simulink library "Simple_lib"  (R2018b)
settings: Solver=ode45  StartTime=0.0  StopTime=10.0  RelTol=1e-3  EnableMultiTasking=on
undefined symbols (not defined in the file or in its folder): Acceptance, beta, C, C_J, C_P, c_wall, dGain, DiscIntNeverNeededParam, Duplex, Electrical_lib, grab, h_fe, i, i3, K_T, Kman, KmanCE, mu_s, n_rev, R_arm, Simplex, systemTs, tau_0, TinIC, Ts, w_0, wallMass, Watch_lib
libraries: $bdroot x407, PlantUtilityBlockset_lib x30, peGeneralControl x22, simulink x11
(part 8 of 14)

== system Simple_lib/Electronics/LR ==
  In1 : Inport
  In2 : Inport  Port=2
  1/R5 : Gain  Gain=-1
  Bus Creator : BusCreator  Inputs=3
  Bus Creator1 : BusCreator  Inputs=3
  Constant : Constant  Value=Phi_0
  Constant1 : Constant  Value=L
  Constant2 : Constant  Value=1/R
  Constant3 : Constant  Value=R
  Ground : Ground
  Ground1 : Ground
  Integrator (Discrete or Continuous) : peGeneralControl/Integrator (Discrete or Continuous)  LabelModeActiveChoice=Discrete  ExternalReset=level  LimitType=Anti-windup  B=inf  A=-inf  Ts=systemTs
  Max : MinMax  Function=max  Inputs=2
  Multiply : Product  Inputs=/*
  Resistance_in : Gain  Gain=R/2
  Resistance_out : Gain  Gain=R/2
  Sum : Sum  Inputs=-|+
  Sum2 : Sum  Inputs=|+-
  Sum3 : Sum  Inputs=|+-
  Weighted Sample Time2 : SampleTimeMath  TsampMathOp=*  weightValue=1
  _in : $bdroot/Electronics/_in  Level=V  Flow=I
      mask init:
      | initInput
      mask Display:
      | % This is a new mask on top of the base mask.
      | % Use "View base mask" link below to see the base mask.
      | %% Icon for flow in
      | % Signally design
      | %plot([0 2 2 3], [1 1 0 0])
      | %plot([1 3 2 1 0 2], [0.6 0.6 0.4 0.6 0.4 0.4])
      | %patch([1 3 2],[0.6 0.6 0.4])
      | %plot([0 1 1], [1 1 0.6])
      | %plot([1 1 0], [0.4 -1 -1])
      | 
      | %color('white')
      | %plot([0 3], [2 2])
      | %plot([0 3], [-2 -2])
      | 
      | %% Bolder design
      | %patch( [0 1 -1], [0 1 1])
      | patch( [-0.1 -0.1 -1], [0.95 0 0.95])
      | patch( [0.1 0.1 1], [1 0 1])
      | plot( [0.1 1 -1 -0.1], [0 -2 -2 0]*0.5)
      | %patch( [-0.1 0.1 0.1 -0.1], [0 0 1 1], [1 1 1])
      | %patch( [-1 0.1 0.1 -1], [1 1 0.95 0.95], [1 1 1])
      | 
      | %% Size the box
      | color('white')
      | plot( [-1 1], [2 2])
      | plot( [-1 1], -[2 2])
  _out : $bdroot/Electronics/_in  Level=V  Flow=I
      mask init:
      | initInput
      mask Display:
      | % This is a new mask on top of the base mask.
      | % Use "View base mask" link below to see the base mask.
      | %% Icon for flow in
      | % Signally design
      | %plot([0 2 2 3], [1 1 0 0])
      | %plot([1 3 2 1 0 2], [0.6 0.6 0.4 0.6 0.4 0.4])
      | %patch([1 3 2],[0.6 0.6 0.4])
      | %plot([0 1 1], [1 1 0.6])
      | %plot([1 1 0], [0.4 -1 -1])
      | 
      | %color('white')
      | %plot([0 3], [2 2])
      | %plot([0 3], [-2 -2])
      | 
      | %% Bolder design
      | %patch( [0 1 -1], [0 1 1])
      | patch( [-0.1 -0.1 -1], [0.95 0 0.95])
      | patch( [0.1 0.1 1], [1 0 1])
      | plot( [0.1 1 -1 -0.1], [0 -2 -2 0]*0.5)
      | %patch( [-0.1 0.1 0.1 -0.1], [0 0 1 1], [1 1 1])
      | %patch( [-1 0.1 0.1 -1], [1 1 0.95 0.95], [1 1 1])
      | 
      | %% Size the box
      | color('white')
      | plot( [-1 1], [2 2])
      | plot( [-1 1], -[2 2])
  wires:
  Weighted Sample Time2/1 -> Max/2  "L_min"
  Constant3/1 -> Weighted Sample Time2/1
  Constant1/1 -> Max/1
  Sum/1 -> Integrator (Discrete or Continuous)/1  "DV"
  Max/1 -> Multiply/1  "L"
  Multiply/1 -> Bus Creator/1, Resistance_out/1, 1/R5/1  "I"
  Bus Creator1/1 -> _in/2
  Bus Creator/1 -> _out/2
  Resistance_out/1 -> Sum3/2
  _out/1 -> Sum3/1
  In2/1 -> _out/1
  Integrator (Discrete or Continuous)/1 -> Multiply/2  "Phi"
  _in/1 -> Sum2/1
  Resistance_in/1 -> Sum2/2
  1/R5/1 -> Resistance_in/1, Bus Creator1/1  "I"
  In1/1 -> _in/1
  Sum2/1 -> Sum/1
  Sum3/1 -> Sum/2
  Constant2/1 -> Bus Creator1/3, Bus Creator/3  "G"
  Ground1/1 -> Bus Creator1/2, Bus Creator/2  "C"
  Constant/1 -> Integrator (Discrete or Continuous)/3
  Ground/1 -> Integrator (Discrete or Continuous)/2

== system Simple_lib/Electronics/M1 ==
  In1 : Inport
  _at : $bdroot/Electronics/_out  Tag=Electrical  Level=V  Flow=I
  _thru : $bdroot/Electronics/_in  Level=V  Flow=I
  Out1 : Outport
  wires:
  _at/1 -> Out1/1
  In1/1 -> _thru/1
  _thru/1 -> _at/1
  _at/2 -> _thru/2

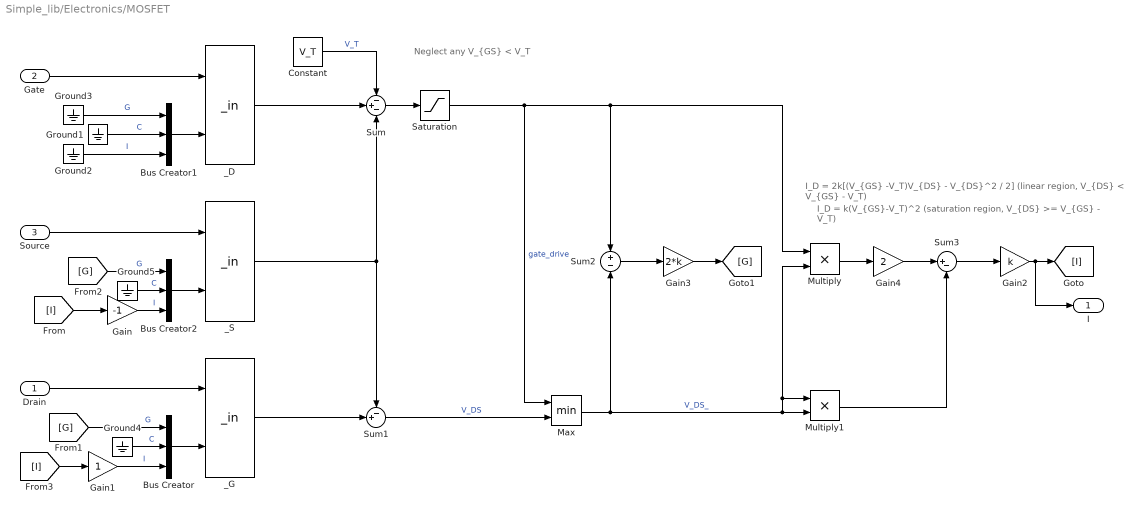
== system Simple_lib/Electronics/MOSFET ==
  note: Neglect any V_{GS} < V_T
  note: I_D = k(V_{GS}-V_T)^2 (saturation region, V_{DS} >= V_{GS} - V_T)
  note: I_D = 2k[(V_{GS} -V_T)V_{DS} - V_{DS}^2 / 2] (linear region, V_{DS} < V_{GS} - V_T)
  Drain : Inport
  Gate : Inport  Port=2
  Source : Inport  Port=3
  Bus Creator : BusCreator  Inputs=3
  Bus Creator1 : BusCreator  Inputs=3
  Bus Creator2 : BusCreator  Inputs=3
  Constant : Constant  Value=V_T
  Gain : Gain  Gain=-1
  Gain1 : Gain
  Gain2 : Gain  Gain=k
  Gain3 : Gain  Gain=2*k
  Gain4 : Gain  Gain=2
  Ground{1..5} (5 alike) : Ground
  Max : MinMax  Inputs=2
  Multiply : Product
  Multiply1 : Product
  Saturation : Saturate  UpperLimit=inf  LowerLimit=0
      settings: AttributesFormatString=|
      | %<UpperLimit>
      | %<LowerLimit>
  Sum : Sum  Inputs=-+-
  Sum1 : Sum  Inputs=-+|
  Sum2 : Sum  Inputs=+|-
  Sum3 : Sum  Inputs=|+-
  _D : $bdroot/Electronics/_in  Level=V  Flow=I
  _G : $bdroot/Electronics/_in  Level=V  Flow=I
  _S : $bdroot/Electronics/_in  Level=V  Flow=I
  I : Outport
  wires:
  Ground5/1 -> Bus Creator2/2  "C"
  Ground4/1 -> Bus Creator/2  "C"
  Gain2/1 -> I/1, [I]
  [I] -> Gain1/1
  [I] -> Gain/1
  [G] -> Bus Creator2/1  "G"
  [G] -> Bus Creator/1  "G"
  Sum3/1 -> Gain2/1
  Gain4/1 -> Sum3/1
  Multiply/1 -> Gain4/1
  Multiply1/1 -> Sum3/2
  Gain3/1 -> [G]
  Sum2/1 -> Gain3/1
  Max/1 -> Multiply/2, Multiply1/1, Multiply1/2, Sum2/2  "V_DS_"
  Sum1/1 -> Max/2  "V_DS"
  Saturation/1 -> Multiply/1, Sum2/1, Max/1  "gate_drive"
  Sum/1 -> Saturation/1
  Constant/1 -> Sum/1  "V_T"
  Ground2/1 -> Bus Creator1/3  "I"
  Gain/1 -> Bus Creator2/3  "I"
  Gain1/1 -> Bus Creator/3  "I"
  Ground3/1 -> Bus Creator1/1  "G"
  Bus Creator2/1 -> _S/2
  Bus Creator1/1 -> _D/2
  Ground1/1 -> Bus Creator1/2  "C"
  Bus Creator/1 -> _G/2
  Source/1 -> _S/1
  _G/1 -> Sum1/2
  _D/1 -> Sum/2
  Drain/1 -> _G/1
  _S/1 -> Sum1/1, Sum/3
  Gate/1 -> _D/1

== system Simple_lib/Electronics/MultiSource ==
  note: The Lump, from which the modelling technique got its name!
      | Lump together all the (grounded) capacitance and use this as inertia term in integrating I to get V.  Q = CV.
      | If there *isn't* much lumpable capacitance attached to this lump then estimate C, knowing R and Ts, by RC = Ts.
      | Integrate the sum of the currents divided by the sum of the grounded capacitances (lumped capacitance) to get the voltage.
      | If there is no capacitance, use Ts * lumped conductance.
  V_in : Inport
  V_in1 : Inport  Port=2
  Abs : Abs
  Abs1 : Abs
  Bus Selector : BusSelector  OutputSignals=I,G,C
  Constant1 : Constant  Value=1/2
  Detect Change : simulink/Logic and Bit Operations/Detect Change  vinit=0  OutDataTypeStr=boolean
  Divide1 : Product  Inputs=*/
  Ground : Ground
  Groundedness (Capacitance to ground) : Constant  Value=V_0
  Integrator (Discrete or Continuous) : peGeneralControl/Integrator (Discrete or Continuous)  LabelModeActiveChoice=Discrete  ExternalReset=level  LimitType=Anti-windup  B=inf  A=-inf  Ts=-1
  Max : MinMax  Function=max  Inputs=3
  Multiply1 : Product  Inputs=3
  Multiply2 : Product
  Saturation : Saturate  UpperLimit=slew_rate  LowerLimit=-slew_rate
      settings: AttributesFormatString=|
      | %<UpperLimit>
      | %<LowerLimit>
  Saturation1 : Saturate  UpperLimit=inf  LowerLimit=1e-12
  Sign convention : Gain  Gain=-1
  Sum : Sum  Inputs=++|
  Terminator1 : Terminator
  Terminator2 : Terminator
  Weighted Sample Time2 : SampleTimeMath  TsampMathOp=*  weightValue=1
  _out : $bdroot/Electronics/_out  Tag=Electrical  Level=V  Flow=I
  out : Outport
  wires:
  Sign convention/1 -> Sum/2  "Current fllow in"
  Saturation1/1 -> Divide1/2, Multiply2/2  "Ceff_sat"
  Integrator (Discrete or Continuous)/1 -> _out/1, Multiply1/1, Multiply2/1  "w"
  Multiply2/1 -> Multiply1/3, Terminator2/1  "conserved_quantity"
  Multiply1/1 -> Terminator1/1  "energy"
  Constant1/1 -> Multiply1/2
  Abs1/1 -> Max/1  "CestPos"
  Abs/1 -> Max/2  "Cpos"
  Sum/1 -> Divide1/1  "Current fllow in"
  Max/1 -> Saturation1/1  "Ceff"
  Weighted Sample Time2/1 -> Abs1/1  "Cest"
  Bus Selector/2 -> Weighted Sample Time2/1  "<G>"
  V_in/1 -> Detect Change/1, Integrator (Discrete or Continuous)/3
  Detect Change/1 -> Integrator (Discrete or Continuous)/2
  Bus Selector/3 -> Abs/1  "<C>"
  Bus Selector/1 -> Sign convention/1  "<I>"
  _out/2 -> Bus Selector/1
  _out/1 -> out/1
  Saturation/1 -> Integrator (Discrete or Continuous)/1  "dV"
  Divide1/1 -> Saturation/1
  Groundedness (Capacitance to ground)/1 -> Max/3
  V_in1/1 -> Sum/1

== system Simple_lib/Electronics/NPN ==
  note: D
  Collector : Inport
  Base : Inport  Port=2
  Emitter : Inport  Port=3
  Dbc : $bdroot/Electronics/D  I_S=1e-12  n=n  T_def=T_def
  Dbe : $bdroot/Electronics/D  I_S=I_S  n=n  T_def=T_def
  Isrc : $bdroot/Electronics/Isrc  SystemSampleTime=-1
  Isrc1 : $bdroot/Electronics/Isrc  SystemSampleTime=-1
  Sum : Sum  Inputs=++|
  Terminator : Terminator
  Terminator1 : Terminator
  alpha_F : Gain  Gain=alpha_F
  alpha_R : Gain  Gain=alpha_R
  I : Outport
  wires:
  Isrc/1 -> Terminator1/1
  Isrc1/1 -> Terminator/1
  Emitter/1 -> Isrc1/1, Dbe/3
  Collector/1 -> Dbc/3, Isrc/1
  Dbc/1 -> Sum/2, [I_BC]  "Icd"
  [I_BE] -> alpha_F/1
  alpha_F/1 -> Sum/1, Isrc/2
  [I_BC] -> alpha_R/1
  alpha_R/1 -> Isrc1/2
  Dbe/1 -> [I_BE]  "Ied"
  Base/1 -> Dbc/1, Isrc/3, Isrc1/3, Dbe/1
  Sum/1 -> I/1

== system Simple_lib/Electronics/NPN_RR ==
  note: D
  Collector : Inport
  Base : Inport  Port=2
  Emitter : Inport  Port=3
  D_Col : $bdroot/Electronics/D_RR  g=1e-3  V_drop=0.6
  D_Emt : $bdroot/Electronics/D_RR  g=1e-3  V_drop=0.6
  Src_Col : $bdroot/Electronics/Isrc  SystemSampleTime=-1
  Src_Emt : $bdroot/Electronics/Isrc  SystemSampleTime=-1
  Terminator : Terminator
  Terminator1 : Terminator
  alpha_F : Gain  Gain=alpha_F
  alpha_R : Gain  Gain=alpha_R
  wires:
  Src_Col/1 -> Terminator1/1
  Src_Emt/1 -> Terminator/1
  Emitter/1 -> D_Emt/2, Src_Emt/1
  Collector/1 -> D_Col/2, Src_Col/1
  D_Col/1 -> [I_CD]  "Icd"
  [I_ED] -> alpha_F/1
  alpha_F/1 -> Src_Col/2
  [I_CD] -> alpha_R/1
  alpha_R/1 -> Src_Emt/2
  D_Emt/1 -> [I_ED]  "Ied"
  Base/1 -> D_Emt/1, D_Col/1, Src_Col/3, Src_Emt/3

== system Simple_lib/Electronics/NPN_SimpleRR ==
  Collector : Inport
  Base : Inport  Port=2
  Emitter : Inport  Port=3
  D_be : $bdroot/Electronics/D_  g_on=0.001  g_off=1e-5  V_drop=1.4
  TransistorMan : Subsystem  mask{V_drop=.6}
      mask prompts: V_drop "Potential Drop (V)"
      mask Display:
      | %patch( [0 -0.05 -0.05 0],[-1 -1 1 1])
      | %patch( [0 1 1],[0 1 -1])
  wires:
  D_be/1 -> TransistorMan/2(I)
  Base/1 -> D_be/1
  Emitter/1 -> TransistorMan/3(Emitter), D_be/2
  Collector/1 -> TransistorMan/1(Collector)

== system Simple_lib/Electronics/OpAmp ==
  note: Just want 1/Ts as the gain, irrespective of the current stuff. I think.
  + : Inport
  - : Inport  Port=2
  Bus Creator1 : BusCreator  Inputs=3
  Ground{,1..4} (5 alike) : Ground
  Integrator (Discrete or Continuous) : peGeneralControl/Integrator (Discrete or Continuous)  LabelModeActiveChoice=Discrete  ExternalReset=level  LimitType=Anti-windup  B=inf  A=-inf  Ts=-1
  Sum : Sum  Inputs=+|-
  Terminator : Terminator
  Weighted Sample Time2 : SampleTimeMath  TsampMathOp=/  weightValue=1
  _out : $bdroot/Electronics/_out  Tag=Electrical  Level=V  Flow=I
  neg : $bdroot/Electronics/OpAmp/pos
      mask init:
      | initInput
      mask Display:
      | % This is a new mask on top of the base mask.
      | % Use "View base mask" link below to see the base mask.
      | %% Icon for flow in
      | % Signally design
      | %plot([0 2 2 3], [1 1 0 0])
      | %plot([1 3 2 1 0 2], [0.6 0.6 0.4 0.6 0.4 0.4])
      | %patch([1 3 2],[0.6 0.6 0.4])
      | %plot([0 1 1], [1 1 0.6])
      | %plot([1 1 0], [0.4 -1 -1])
      | 
      | %color('white')
      | %plot([0 3], [2 2])
      | %plot([0 3], [-2 -2])
      | 
      | %% Bolder design
      | %patch( [0 1 -1], [0 1 1])
      | patch( [-0.1 -0.1 -1], [0.95 0 0.95])
      | patch( [0.1 0.1 1], [1 0 1])
      | plot( [0.1 1 -1 -0.1], [0 -2 -2 0]*0.5)
      | %patch( [-0.1 0.1 0.1 -0.1], [0 0 1 1], [1 1 1])
      | %patch( [-1 0.1 0.1 -1], [1 1 0.95 0.95], [1 1 1])
      | 
      | %% Size the box
      | color('white')
      | plot( [-1 1], [2 2])
      | plot( [-1 1], -[2 2])
  pos : $bdroot/Electronics/_in  Level=V  Flow=I
      mask init:
      | initInput
      mask Display:
      | % This is a new mask on top of the base mask.
      | % Use "View base mask" link below to see the base mask.
      | %% Icon for flow in
      | % Signally design
      | %plot([0 2 2 3], [1 1 0 0])
      | %plot([1 3 2 1 0 2], [0.6 0.6 0.4 0.6 0.4 0.4])
      | %patch([1 3 2],[0.6 0.6 0.4])
      | %plot([0 1 1], [1 1 0.6])
      | %plot([1 1 0], [0.4 -1 -1])
      | 
      | %color('white')
      | %plot([0 3], [2 2])
      | %plot([0 3], [-2 -2])
      | 
      | %% Bolder design
      | %patch( [0 1 -1], [0 1 1])
      | patch( [-0.1 -0.1 -1], [0.95 0 0.95])
      | patch( [0.1 0.1 1], [1 0 1])
      | plot( [0.1 1 -1 -0.1], [0 -2 -2 0]*0.5)
      | %patch( [-0.1 0.1 0.1 -0.1], [0 0 1 1], [1 1 1])
      | %patch( [-1 0.1 0.1 -1], [1 1 0.95 0.95], [1 1 1])
      | 
      | %% Size the box
      | color('white')
      | plot( [-1 1], [2 2])
      | plot( [-1 1], -[2 2])
  Out1 : Outport
  wires:
  _out/2 -> Terminator/1
  Ground2/1 -> Integrator (Discrete or Continuous)/3
  Ground/1 -> Integrator (Discrete or Continuous)/2
  pos/1 -> Sum/1
  neg/1 -> Sum/2
  +/1 -> pos/1
  -/1 -> neg/1
  _out/1 -> Out1/1
  Sum/1 -> Weighted Sample Time2/1
  Integrator (Discrete or Continuous)/1 -> _out/1
  Weighted Sample Time2/1 -> Integrator (Discrete or Continuous)/1
  Bus Creator1/1 -> neg/2, pos/2
  Ground4/1 -> Bus Creator1/2  "C"
  Ground3/1 -> Bus Creator1/1  "I"
  Ground1/1 -> Bus Creator1/3  "G"

== system Simple_lib/Electronics/PNP ==
  note: D
  Collector : Inport
  Base : Inport  Port=2
  Emitter : Inport  Port=3
  Dbc : $bdroot/Electronics/D  I_S=1e-12  n=1  T_def=300
  Dbe : $bdroot/Electronics/D  I_S=1e-12  n=1  T_def=300
  Isrc : $bdroot/Electronics/Isrc  SystemSampleTime=-1
  Isrc1 : $bdroot/Electronics/Isrc  SystemSampleTime=-1
  Sum : Sum  Inputs=++|
  Terminator : Terminator
  Terminator1 : Terminator
  alpha_F : Gain  Gain=alpha_F
  alpha_R : Gain  Gain=alpha_R
  I : Outport
  wires:
  Isrc1/1 -> Terminator1/1
  Isrc/1 -> Terminator/1
  Emitter/1 -> Dbe/1, Isrc/3
  Collector/1 -> Isrc1/3, Dbc/1
  [I_EB] -> alpha_F/1
  [I_CB] -> alpha_R/1
  alpha_R/1 -> Isrc/2
  Dbe/1 -> [I_EB]  "Ied"
  Base/1 -> Dbc/3, Dbe/3, Isrc1/1, Isrc/1
  Dbc/1 -> Sum/2, [I_CB]  "Icd"
  alpha_F/1 -> Isrc1/2, Sum/1
  Sum/1 -> I/1

== system Simple_lib/Electronics/PNP_RR ==
  note: D
  Collector : Inport
  Base : Inport  Port=2
  Emitter : Inport  Port=3
  D_bc : $bdroot/Electronics/D_RR  g=1e-3  V_drop=0.6
  D_be : $bdroot/Electronics/D_RR  g=1e-3  V_drop=0.6
  Isrc : $bdroot/Electronics/Isrc  SystemSampleTime=-1
  Isrc1 : $bdroot/Electronics/Isrc  SystemSampleTime=-1
  Terminator : Terminator
  Terminator1 : Terminator
  alpha_F : Gain  Gain=alpha_F
  alpha_R : Gain  Gain=alpha_R
  wires:
  Isrc1/1 -> Terminator1/1
  Isrc/1 -> Terminator/1
  Emitter/1 -> D_be/1, Isrc/3
  Collector/1 -> D_bc/1, Isrc1/3
  D_bc/1 -> [I_CD]  "Icd"
  [I_ED] -> alpha_F/1
  alpha_F/1 -> Isrc1/2
  [I_CD] -> alpha_R/1
  alpha_R/1 -> Isrc/2
  D_be/1 -> [I_ED]  "Ied"
  Base/1 -> D_bc/2, D_be/2, Isrc1/1, Isrc/1

== system Simple_lib/Electronics/Q ==
  Collector : Inport
  Emitter : Inport  Port=2
  Diode : $bdroot/Electronics/Reverse  V_drop=0
  Sum : Sum  Inputs=+|+
  TransAction : $bdroot/Electronics/TransAction  V_drop=.6
  Base : Outport
  wires:
  TransAction/1 -> Sum/1
  Sum/1 -> Base/1
  Collector/1 -> TransAction/1
  Emitter/1 -> Diode/1
  Diode/1 -> TransAction/2, Sum/2

== system Simple_lib/Electronics/Q1 ==
  note: D
  Collector : Inport
  Base : Inport  Port=2
  Emitter : Inport  Port=3
  Dc : $bdroot/Electronics/D_  g_on=g_on  g_off=g_off  V_drop=V_drop
  De : $bdroot/Electronics/D_  g_on=1e-1  g_off=0  V_drop=0.6
  Ic : $bdroot/Electronics/Isrc  SystemSampleTime=-1
  Ie : $bdroot/Electronics/Isrc  SystemSampleTime=-1
  Terminator : Terminator
  Terminator1 : Terminator
  alpha_F : Gain  Gain=alpha_F
  alpha_R : Gain  Gain=alpha_R
  wires:
  Base/1 -> De/1, Dc/1, Ie/3, Ic/3
  De/1 -> alpha_F/1  "Ied"
  alpha_R/1 -> Ie/2
  alpha_F/1 -> Ic/2
  Dc/1 -> alpha_R/1  "Icd"
  Collector/1 -> Dc/2, Ic/1
  Emitter/1 -> De/2, Ie/1
  Ie/1 -> Terminator/1
  Ic/1 -> Terminator1/1

== system Simple_lib/Electronics/Q2 ==
  note: D
  Collector : Inport
  Base : Inport  Port=2
  Emitter : Inport  Port=3
  Dc : $bdroot/Electronics/D_  g_on=0.001  g_off=1e-5  V_drop=V_drop
  De : $bdroot/Electronics/D_  g_on=0.001  g_off=1e-5  V_drop=V_drop
  Isrc : $bdroot/Electronics/Isrc  SystemSampleTime=-1
  Isrc1 : $bdroot/Electronics/Isrc  SystemSampleTime=-1
  Terminator : Terminator
  Terminator1 : Terminator
  alpha_F : Gain  Gain=alpha_F
  alpha_R : Gain  Gain=alpha_R
  wires:
  Isrc1/1 -> Terminator1/1
  Isrc/1 -> Terminator/1
  Emitter/1 -> De/1, Isrc/3
  Collector/1 -> Dc/1, Isrc1/3
  Dc/1 -> alpha_R/1  "Icd"
  alpha_F/1 -> Isrc1/2
  alpha_R/1 -> Isrc/2
  De/1 -> alpha_F/1  "Ied"
  Base/1 -> De/2, Dc/2, Isrc1/1, Isrc/1

== system Simple_lib/Electronics/Q_NPN ==
  note: D
  Base : Inport
  Ammeter : $bdroot/Electronics/Ammeter  SystemSampleTime=-1
  Ammeter1 : $bdroot/Electronics/Ammeter  SystemSampleTime=-1
  Dbc : $bdroot/Electronics/Forward  V_drop=0.6
  Dbe : $bdroot/Electronics/Forward  V_drop=0.6
  SrcCb : $bdroot/Electronics/Isrc  SystemSampleTime=-1
  SrcEb : $bdroot/Electronics/Isrc  SystemSampleTime=-1
  Sum : Sum  Inputs=++|
  Sum1 : Sum  Inputs=++|
  Terminator : Terminator
  Terminator1 : Terminator
  Unit Delay1 : UnitDelay  SampleTime=-1
  Unit Delay2 : UnitDelay  Commented=through  SampleTime=-1
  alpha_F : Gain  Gain=alpha_F
  alpha_R : Gain  Gain=alpha_R
  C : Outport
  E : Outport  Port=2
  wires:
  Unit Delay2/1 -> SrcEb/2
  Unit Delay1/1 -> SrcCb/2
  alpha_R/1 -> Unit Delay2/1
  Ammeter1/1 -> Sum/1
  Ammeter/1 -> Sum1/1
  Dbe/1 -> Sum/2
  Dbc/1 -> Sum1/2
  Base/1 -> Dbc/1, Dbe/1, SrcCb/3, SrcEb/3
  SrcCb/1 -> Terminator1/1
  SrcEb/1 -> Terminator/1
  Sum/1 -> E/1, SrcEb/1
  Sum1/1 -> SrcCb/1, C/1
  Ammeter/2 -> alpha_R/1  "Ibc"
  alpha_F/1 -> Unit Delay1/1
  Ammeter1/2 -> alpha_F/1  "Ibe"

== system Simple_lib/Electronics/R ==
  pos : Inport
  neg : Inport  Port=2
  1/R1 : Gain  Gain=-1
  Bus Creator : BusCreator  Inputs=3
  Bus Creator1 : BusCreator  Inputs=3
  Constant1 : Constant  Value=1/R
  Ground : Ground
  Sum : Sum  Inputs=+|-
  _neg : $bdroot/Electronics/_in  Level=V  Flow=I
  _pos : $bdroot/Electronics/_in  Level=V  Flow=I
  conductance1 : Gain  Gain=1/R
  I : Outport
  wires:
  _neg/1 -> Sum/2
  1/R1/1 -> Bus Creator1/3  "I"
  conductance1/1 -> Bus Creator/1, I/1, 1/R1/1  "I"
  Bus Creator/1 -> _pos/2
  Sum/1 -> conductance1/1
  Bus Creator1/1 -> _neg/2
  _pos/1 -> Sum/1
  pos/1 -> _pos/1
  neg/1 -> _neg/1
  Constant1/1 -> Bus Creator/2, Bus Creator1/2  "G"
  Ground/1 -> Bus Creator1/1, Bus Creator/3  "C"

== system Simple_lib/Electronics/R1 ==
  pos : Inport
  neg : Inport  Port=2
  1/R1 : Gain  Gain=-1
  Bus Creator : BusCreator  Inputs=3
  Bus Creator1 : BusCreator  Inputs=3
  Constant1 : Constant  Value=1/R
  Ground : Ground
  Sum : Sum  Inputs=+|-
  _neg : $bdroot/Electronics/_in  Level=V  Flow=I
  _pos : $bdroot/Electronics/_in  Level=V  Flow=I
  conductance1 : Gain  Gain=1/R
  I : Outport
  wires:
  _neg/1 -> Sum/2
  1/R1/1 -> Bus Creator1/3  "I"
  conductance1/1 -> Bus Creator/1, I/1, 1/R1/1  "I"
  Bus Creator/1 -> _pos/2
  Sum/1 -> conductance1/1
  Bus Creator1/1 -> _neg/2
  _pos/1 -> Sum/1
  pos/1 -> _pos/1
  neg/1 -> _neg/1
  Constant1/1 -> Bus Creator/2, Bus Creator1/2  "G"
  Ground/1 -> Bus Creator1/1, Bus Creator/3  "C"

== system Simple_lib/Electronics/R_ ==
  In1 : Inport
  Ground1 : Ground
  at : $bdroot/Electronics/TP  V_0=0  slew_rate=1000  conserved_quantity_name=Q  energy_name=E
  thru : $bdroot/Electronics/R  R=R
      settings: AttributesFormatString=%<R> Ohms
  Out1 : Outport
  wires:
  In1/1 -> thru/1
  at/1 -> thru/2, Out1/1
  Ground1/1 -> at/1

== system Simple_lib/Electronics/R_1 ==
  In1 : Inport
  Bus Selector : BusSelector  OutputSignals=I
  In : $bdroot/Electronics/_in  Level=V  Flow=I
      mask init:
      | initInput
      mask Display:
      | % This is a new mask on top of the base mask.
      | % Use "View base mask" link below to see the base mask.
      | %% Icon for flow in
      | % Signally design
      | %plot([0 2 2 3], [1 1 0 0])
      | %plot([1 3 2 1 0 2], [0.6 0.6 0.4 0.6 0.4 0.4])
      | %patch([1 3 2],[0.6 0.6 0.4])
      | %plot([0 1 1], [1 1 0.6])
      | %plot([1 1 0], [0.4 -1 -1])
      | 
      | %color('white')
      | %plot([0 3], [2 2])
      | %plot([0 3], [-2 -2])
      | 
      | %% Bolder design
      | %patch( [0 1 -1], [0 1 1])
      | patch( [-0.1 -0.1 -1], [0.95 0 0.95])
      | patch( [0.1 0.1 1], [1 0 1])
      | plot( [0.1 1 -1 -0.1], [0 -2 -2 0]*0.5)
      | %patch( [-0.1 0.1 0.1 -0.1], [0 0 1 1], [1 1 1])
      | %patch( [-1 0.1 0.1 -1], [1 1 0.95 0.95], [1 1 1])
      | 
      | %% Size the box
      | color('white')
      | plot( [-1 1], [2 2])
      | plot( [-1 1], -[2 2])
  Sum : Sum  Inputs=|+-
  _out : $bdroot/Electronics/_out  Tag=Electrical  Level=V  Flow=I
  resistance : Gain  Gain=R
  Out1 : Outport
  wires:
  In/1 -> Sum/1
  _out/2 -> In/2, Bus Selector/1
  resistance/1 -> Sum/2
  Sum/1 -> _out/1
  _out/1 -> Out1/1
  In1/1 -> In/1
  Bus Selector/1 -> resistance/1  "<I>"

== system Simple_lib/Electronics/R_Gnd ==
  In1 : Inport
  Gnd : $bdroot/Electronics/Earth  SystemSampleTime=-1
  at : $bdroot/Electronics/R  R=R
      settings: AttributesFormatString=%<R> Ohms
  wires:
  In1/1 -> at/1
  Gnd/1 -> at/2

== system Simple_lib/Electronics/Rail ==
  V : Inport
  Bus Selector : BusSelector  OutputSignals=I
  Constant : Constant  Value=Vcc
  Sum : Sum  Inputs=|++
  _in : $bdroot/Electronics/_out  Tag=Electrical  Level=V  Flow=I
  I : Outport
  Vcc : Outport  Port=2
  wires:
  _in/1 -> Vcc/1
  Constant/1 -> Sum/2
  _in/2 -> Bus Selector/1
  Bus Selector/1 -> I/1  "<I>"
  Sum/1 -> _in/1
  V/1 -> Sum/1

== system Simple_lib/Electronics/ResistiveSwitch ==
  s : Inport
  In2 : Inport  Port=2
  Switch : $bdroot/Electronics/Switch  SystemSampleTime=-1
  from : $bdroot/Electronics/TP  V_0=0  slew_rate=100.0  conserved_quantity_name=Q  energy_name=E
  Out1 : Outport
  wires:
  In2/1 -> Switch/3
  from/1 -> Switch/1, Out1/1
  s/1 -> Switch/2

== system Simple_lib/Electronics/Reverse ==
  in : Inport
  Bus Creator2 : BusCreator  Inputs=3
  Bus Selector : BusSelector  OutputSignals=I,C,G
  Bus Selector1 : BusSelector  OutputSignals=I,C,G
  Constant : Constant  Value=-V_drop
  Divide1 : Product  Inputs=*/
  Gain : Gain
  Gain1 : Gain
  Ground : Ground
  Ground1 : Ground  Commented=on
  Integrator (Discrete or Continuous) : peGeneralControl/Integrator (Discrete or Continuous)  LabelModeActiveChoice=Discrete  ExternalReset=level  LimitType=Anti-windup  B=inf  A=-V_drop  Ts=systemTs
  Sum1 : Sum  Inputs=|+-
  Switch : Switch  Criteria=u2 ~= 0
  Weighted Sample Time : SampleTimeMath  TsampMathOp=*
  _in : $bdroot/Electronics/_in  Level=V  Flow=I
  _out : $bdroot/Electronics/_out  Tag=Electrical  Level=V  Flow=I
  out : Outport
  wires:
  Bus Creator2/1 -> _in/2
  Gain1/1 -> Bus Creator2/2  "C"
  Gain/1 -> Bus Creator2/3  "G"
  Bus Selector1/3 -> Gain/1  "<G>"
  Bus Selector1/2 -> Gain1/1  "<C>"
  Bus Selector1/1 -> Bus Creator2/1  "<I>"
  Ground1/1 -> ?  "I"
  _out/1 -> out/1
  Integrator (Discrete or Continuous)/1 -> Sum1/2
  _in/1 -> Sum1/1
  in/1 -> _in/1
  Sum1/1 -> _out/1
  Bus Selector/2 -> Switch/1, Switch/2  "<C>"
  Bus Selector/1 -> Divide1/1  "<I>"
  Divide1/1 -> Integrator (Discrete or Continuous)/1
  Constant/1 -> Integrator (Discrete or Continuous)/3
  Ground/1 -> Integrator (Discrete or Continuous)/2
  _out/2 -> Bus Selector/1, Bus Selector1/1
  Weighted Sample Time/1 -> Switch/3
  Bus Selector/3 -> Weighted Sample Time/1  "<G>"
  Switch/1 -> Divide1/2

== system Simple_lib/Electronics/Rnl1 ==
  note: Put the exponential terms from Ebers Moll in here - the Shockley model
  pos : Inport
  neg : Inport  Port=2
  1/R1 : Gain  Gain=-1
  Bus Creator : BusCreator  Inputs=3
  Bus Creator1 : BusCreator  Inputs=3
  Derivative : Subsystem
  Ground : Ground
  I/V curve : Lookup_n-D  Commented=on  NumberOfTableDimensions=1  BreakpointsForDimension1=[-5:5]  Table=tanh([-5:5])  InternalRulePriority=Speed  RndMeth=Simplest  InputSameDT=on
  I/V curve1 : Lookup_n-D  NumberOfTableDimensions=1  BreakpointsForDimension1=[-5:5]  Table=[0 0 0 0 0 0 0 1 10 100 1000]  InternalRulePriority=Speed  RndMeth=Simplest  InputSameDT=on
  Sum : Sum  Inputs=+|-
  _neg : $bdroot/Electronics/_in  Level=V  Flow=I
      mask init:
      | initInput
      mask Display:
      | % This is a new mask on top of the base mask.
      | % Use "View base mask" link below to see the base mask.
      | %% Icon for flow in
      | % Signally design
      | %plot([0 2 2 3], [1 1 0 0])
      | %plot([1 3 2 1 0 2], [0.6 0.6 0.4 0.6 0.4 0.4])
      | %patch([1 3 2],[0.6 0.6 0.4])
      | %plot([0 1 1], [1 1 0.6])
      | %plot([1 1 0], [0.4 -1 -1])
      | 
      | %color('white')
      | %plot([0 3], [2 2])
      | %plot([0 3], [-2 -2])
      | 
      | %% Bolder design
      | %patch( [0 1 -1], [0 1 1])
      | patch( [-0.1 -0.1 -1], [0.95 0 0.95])
      | patch( [0.1 0.1 1], [1 0 1])
      | plot( [0.1 1 -1 -0.1], [0 -2 -2 0]*0.5)
      | %patch( [-0.1 0.1 0.1 -0.1], [0 0 1 1], [1 1 1])
      | %patch( [-1 0.1 0.1 -1], [1 1 0.95 0.95], [1 1 1])
      | 
      | %% Size the box
      | color('white')
      | plot( [-1 1], [2 2])
      | plot( [-1 1], -[2 2])
  _pos : $bdroot/Electronics/_in  Level=V  Flow=I
      mask init:
      | initInput
      mask Display:
      | % This is a new mask on top of the base mask.
      | % Use "View base mask" link below to see the base mask.
      | %% Icon for flow in
      | % Signally design
      | %plot([0 2 2 3], [1 1 0 0])
      | %plot([1 3 2 1 0 2], [0.6 0.6 0.4 0.6 0.4 0.4])
      | %patch([1 3 2],[0.6 0.6 0.4])
      | %plot([0 1 1], [1 1 0.6])
      | %plot([1 1 0], [0.4 -1 -1])
      | 
      | %color('white')
      | %plot([0 3], [2 2])
      | %plot([0 3], [-2 -2])
      | 
      | %% Bolder design
      | %patch( [0 1 -1], [0 1 1])
      | patch( [-0.1 -0.1 -1], [0.95 0 0.95])
      | patch( [0.1 0.1 1], [1 0 1])
      | plot( [0.1 1 -1 -0.1], [0 -2 -2 0]*0.5)
      | %patch( [-0.1 0.1 0.1 -0.1], [0 0 1 1], [1 1 1])
      | %patch( [-1 0.1 0.1 -1], [1 1 0.95 0.95], [1 1 1])
      | 
      | %% Size the box
      | color('white')
      | plot( [-1 1], [2 2])
      | plot( [-1 1], -[2 2])
  I : Outport
  wires:
  1/R1/1 -> Bus Creator1/2  "I"
  Bus Creator/1 -> _pos/2
  Derivative/1(dy/dx) -> Bus Creator/1, Bus Creator1/3  "G"
  pos/1 -> _pos/1
  _pos/1 -> Sum/1
  Sum/1 -> I/V curve1/1, Derivative/2(x)  "D_V"
  neg/1 -> _neg/1
  _neg/1 -> Sum/2
  I/V curve1/1 -> I/1, 1/R1/1, Bus Creator/2, Derivative/1(y)  "I"
  Bus Creator1/1 -> _neg/2
  Ground/1 -> Bus Creator/3, Bus Creator1/1  "C"

== system Simple_lib/Electronics/Switch ==
  In1 : Inport
  In2 : Inport  Port=2
  In3 : Inport  Port=3
  Switch : Switch  Criteria=u2 ~= 0
  VR : $bdroot/Electronics/VR  SystemSampleTime=-1
  g_off : Constant  Value=10e-9
  g_on : Constant  Value=100
  wires:
  In2/1 -> Switch/2
  In3/1 -> VR/3
  In1/1 -> VR/1
  Switch/1 -> VR/2
  g_on/1 -> Switch/1
  g_off/1 -> Switch/3

== system Simple_lib/Electronics/Switch2 ==
  In1 : Inport
  In2 : Inport  Port=2
  In3 : Inport  Port=3
  Ground : Ground
  Ground1 : Ground
  Switch : Switch  Criteria=u2 ~= 0
  Switch1 : Switch  Criteria=u2 ~= 0
  Switch2 : Switch  Criteria=u2 ~= 0
  _in1 : $bdroot/Electronics/_in  Level=V  Flow=I
  _in2 : $bdroot/Electronics/_in  Level=V  Flow=I
  _out : $bdroot/Electronics/_out  Tag=Electrical  Level=V  Flow=I
  Output : Outport
  wires:
  In2/1 -> Switch1/2, Switch2/2, Switch/2
  In3/1 -> _in2/1
  In1/1 -> _in1/1
  Switch/1 -> _out/1
  _in1/1 -> Switch/1
  _in2/1 -> Switch/3
  _out/1 -> Output/1
  _out/2 -> [I]
  Switch2/1 -> _in2/2
  Switch1/1 -> _in1/2
  [I] -> Switch1/1
  [I] -> Switch2/3
  Ground1/1 -> Switch2/1
  Ground/1 -> Switch1/3

== system Simple_lib/Electronics/TP ==
  note: The Lump, from which the modelling technique got its name!
      | Lump together all the (grounded) capacitance and use this as inertia term in integrating I to get V.  Q = CV.
      | If there *isn't* much lumpable capacitance attached to this lump then estimate C, knowing R and Ts, by RC = Ts.
      | Integrate the sum of the currents divided by the sum of the grounded capacitances (lumped capacitance) to get the voltage.
      | If there is no capacitance, use Ts * lumped conductance.
  I : Inport
  Abs : Abs
  Abs1 : Abs
  Bus Selector : BusSelector  OutputSignals=I,G,C
  Constant : Constant  Value=V_0
  Constant1 : Constant  Value=1/2
  Divide1 : Product  Inputs=*/
  Ground : Ground
  Integrator (Discrete or Continuous) : peGeneralControl/Integrator (Discrete or Continuous)  LabelModeActiveChoice=Discrete  ExternalReset=level  LimitType=Anti-windup  B=inf  A=-inf  Ts=-1
  Max : MinMax  Function=max  Inputs=2
  Multiply1 : Product  Inputs=3
  Multiply2 : Product
  Saturation : Saturate  UpperLimit=slew_rate  LowerLimit=-slew_rate
      settings: AttributesFormatString=|
      | %<UpperLimit>
      | %<LowerLimit>
  Saturation1 : Saturate  UpperLimit=inf  LowerLimit=1e-12
  Sign convention : Gain  Gain=-1
  Sum : Sum  Inputs=++|
  Terminator1 : Terminator
  Terminator2 : Terminator
  Weighted Sample Time2 : SampleTimeMath  TsampMathOp=*  weightValue=1
  _out : $bdroot/Electronics/_out  Tag=Electrical  Level=V  Flow=I
  out : Outport
  wires:
  Divide1/1 -> Saturation/1
  Saturation/1 -> Integrator (Discrete or Continuous)/1  "dV"
  _out/1 -> out/1
  _out/2 -> Bus Selector/1
  Bus Selector/1 -> Sign convention/1  "<I>"
  Bus Selector/3 -> Abs/1  "C"
  Ground/1 -> Integrator (Discrete or Continuous)/2
  Constant/1 -> Integrator (Discrete or Continuous)/3
  Bus Selector/2 -> Weighted Sample Time2/1  "<G>"
  Weighted Sample Time2/1 -> Abs1/1  "Cest"
  Max/1 -> Saturation1/1  "Ceff"
  Sum/1 -> Divide1/1  "Current fllow in"
  Abs/1 -> Max/2  "Cpos"
  Abs1/1 -> Max/1  "CestPos"
  Constant1/1 -> Multiply1/2
  Multiply1/1 -> Terminator1/1  "energy"
  Multiply2/1 -> Terminator2/1, Multiply1/3  "conserved_quantity"
  Integrator (Discrete or Continuous)/1 -> Multiply2/1, Multiply1/1, _out/1  "w"
  Saturation1/1 -> Multiply2/2, Divide1/2  "Jeff_sat"
  I/1 -> Sum/1
  Sign convention/1 -> Sum/2  "Current fllow in"

== system Simple_lib/Electronics/TransAction ==
  Collector : Inport
  Emitter : Inport  Port=2
  Bus Creator : BusCreator  Inputs=3
  Bus Creator1 : BusCreator  Inputs=3
  Bus Selector : BusSelector  OutputSignals=I
  Constant : Constant  Value=99
  Constant1 : Constant  Value=99
  Cosh : Trigonometry  Operator=cosh
  Gain : Gain  Gain=-1
  Gain1 : Gain  Gain=-1
  Gain2 : Gain
  Gain3 : Gain
  Ground : Ground
  Ground1 : Ground
  Multiply : Product  Inputs=3
  Multiply1 : Product  Inputs=*//*
  Saturation : Saturate  UpperLimit=inf  LowerLimit=-inf
  Sum : Sum  Inputs=+|-
  Tanh : Trigonometry  Operator=tanh
  _Base : $bdroot/Electronics/_out  Tag=Electrical  Level=V  Flow=I
  _Col : $bdroot/Electronics/_in  Level=V  Flow=I
  _Em : $bdroot/Electronics/_in  Level=V  Flow=I
  Dummy : Outport
  wires:
  Gain3/1 -> Bus Creator/1  "I"
  Gain2/1 -> Bus Creator1/2  "G"
  Gain1/1 -> Saturation/1  "I"
  Saturation/1 -> Multiply/1, Multiply1/4
  Bus Selector/1 -> Gain1/1  "<I>"
  Constant1/1 -> Multiply1/1
  Multiply1/1 -> Bus Creator/2, Gain2/1  "G"
  Cosh/1 -> Multiply1/3, Multiply1/2
  Bus Creator/1 -> _Col/2
  Bus Creator1/1 -> _Em/2
  Ground1/1 -> Bus Creator/3, Bus Creator1/1  "C"
  Gain/1 -> Bus Creator1/3  "I"
  Multiply/1 -> Gain/1, Gain3/1  "I"
  Constant/1 -> Multiply/3
  _Base/2 -> Bus Selector/1
  Tanh/1 -> Multiply/2
  Sum/1 -> Tanh/1, Cosh/1
  _Em/1 -> Sum/2
  Emitter/1 -> _Em/1
  _Base/1 -> Dummy/1
  _Col/1 -> Sum/1
  Collector/1 -> _Col/1
  Ground/1 -> _Base/1

== system Simple_lib/Electronics/VR ==
  pos : Inport
  G : Inport  Port=2
  neg : Inport  Port=3
  1/R1 : Gain  Gain=-1
  Bus Creator2 : BusCreator  Inputs=3
  Bus Creator3 : BusCreator  Inputs=3
  Bus Selector : BusSelector  OutputSignals=I
  Ground : Ground
  Multiply : Product
  Multiply1 : Product
  Sum : Sum  Inputs=+|-
  _neg : $bdroot/Electronics/_in  Level=V  Flow=I
  _pos : $bdroot/Electronics/_in  Level=V  Flow=I
  I : Outport
  wires:
  _neg/1 -> Sum/2
  1/R1/1 -> Bus Creator3/3  "I"
  Sum/1 -> Multiply/1, Multiply1/2  "DV"
  Bus Creator2/1 -> Bus Selector/1, _pos/2
  Bus Creator3/1 -> _neg/2
  _pos/1 -> Sum/1
  pos/1 -> _pos/1
  neg/1 -> _neg/1
  G/1 -> Bus Creator2/2, Bus Creator3/2, Multiply/2, Multiply1/1  "G"
  Multiply1/1 -> 1/R1/1
  Ground/1 -> Bus Creator3/1, Bus Creator2/3  "C"
  Multiply/1 -> Bus Creator2/1  "I"
  Bus Selector/1 -> I/1  "<I>"

== system Simple_lib/Electronics/VoltMeter ==
  V_in : Inport
  Terminator : Terminator
  _out : $bdroot/Electronics/_out  Tag=Electrical  Level=V  Flow=I
  V_sys : Outport
  wires:
  _out/1 -> V_sys/1
  _out/2 -> Terminator/1
  V_in/1 -> _out/1

== system Simple_lib/Electronics/VoltageSource ==
  V_in : Inport
  Terminator : Terminator
  _out : $bdroot/Electronics/_out  Tag=Electrical  Level=V  Flow=I
  V_sys : Outport
  wires:
  _out/1 -> V_sys/1
  _out/2 -> Terminator/1
  V_in/1 -> _out/1

== system Simple_lib/Electronics/_in ==
  note: {\bf\_in - wraps up the {\itInflow} block}
      |
      | The init function {\itinit\_in} sets up the logging of the level and flow names.
  in : Inport
  back : Inport  Port=2
  Bus Selector : BusSelector  OutputSignals=I,G,C
  Constant : Constant  Value=[0,0,0]
  Inflow : $bdroot/Utility/Inflow  SystemSampleTime=-1
  Mux : Mux  Inputs=3
  Sum : Sum  Inputs=|++
  out : Outport
  wires:
  Constant/1 -> Sum/2
  Sum/1 -> Inflow/2
  Bus Selector/2 -> Mux/2  "<G>"
  in/1 -> Inflow/1  "V"
  back/1 -> Bus Selector/1
  Bus Selector/3 -> Mux/3  "<C>"
  Bus Selector/1 -> Mux/1  "<I>"
  Inflow/1 -> out/1
  Mux/1 -> Sum/1

== system Simple_lib/Electronics/_out ==
  note: {\bf\_out - buses out and logs the signals from the generic {\itOutflow} block}
      |
      | The init function {\itinit\_out} sets up the logging.
  in : Inport  Tag=NOFLUX
  Bus Creator : BusCreator  Inputs=3
  Demux : Demux  Outputs=3
  Outflow : $bdroot/Utility/Outflow  Tag=Electrical  SystemSampleTime=-1
  Reassure Simulink about the dimensionality! : Constant  Value=[0;0;0]
  Sum : Sum  Inputs=|++
  Sum2 : Sum  Inputs=+  CollapseMode=Specified dimension  CollapseDim=2
  out : Outport
  backs : Outport  Tag=NOFLUX  Port=2
  wires:
  Reassure Simulink about the dimensionality!/1 -> Sum/2
  Sum/1 -> Demux/1
  Sum2/1 -> Sum/1
  Demux/2 -> Bus Creator/2  "G"
  Demux/1 -> Bus Creator/1  "I"
  Outflow/2 -> Sum2/1
  in/1 -> Outflow/1  "V"
  Bus Creator/1 -> backs/1
  Outflow/1 -> out/1
  Demux/3 -> Bus Creator/3  "C"

== system Simple_lib/Electronics/badQ ==
  note: D
  Collector : Inport
  Base : Inport  Port=2
  Emitter : Inport  Port=3
  D_Col : $bdroot/Electronics/D_  g_on=0.01  g_off=1e-5  V_drop=0.6
  D_Emt : $bdroot/Electronics/D_  g_on=0.01  g_off=1e-5  V_drop=0.6
  Src_Col : $bdroot/Electronics/Isrc  SystemSampleTime=-1
  Src_Emt : $bdroot/Electronics/Isrc  SystemSampleTime=-1
  Terminator : Terminator
  Terminator1 : Terminator
  alpha_F : Gain  Gain=alpha_F
  alpha_R : Gain  Gain=alpha_R
  wires:
  Base/1 -> D_Col/1, D_Emt/1, Src_Emt/3, Src_Col/3
  D_Emt/1 -> [I_ED]  "Ied"
  alpha_R/1 -> Src_Emt/2
  [I_CD] -> alpha_R/1
  alpha_F/1 -> Src_Col/2
  [I_ED] -> alpha_F/1
  D_Col/1 -> [I_CD]  "Icd"
  Collector/1 -> D_Col/2, Src_Col/1
  Emitter/1 -> D_Emt/2, Src_Emt/1
  Src_Emt/1 -> Terminator/1
  Src_Col/1 -> Terminator1/1

== system Simple_lib/Electronics/bigain ==
  In1 : Inport
  Duplex : $bdroot/Electronics/_out  Tag=Electrical  Level=Level  Flow=flow
  Simplex : $bdroot/Electronics/_in  Tag=Electrical  Level=V  Flow=I
  h_fe : Gain  Gain=100
  h_re : Gain  Gain=1e-6
  Out1 : Outport
  wires:
  Duplex/1 -> Out1/1
  Simplex/1 -> h_re/1
  In1/1 -> Simplex/1
  h_fe/1 -> Simplex/2
  h_re/1 -> Duplex/1
  Duplex/2 -> h_fe/1

== system Simple_lib/Hydraulic/ Heat Exchanger ==
  in1 : Inport
  in2 : Inport  Port=2
  Bus Creator : BusCreator  Inputs=2
  Bus Creator1 : BusCreator  Inputs=2
  Bus Selector : BusSelector  OutputSignals=p,T
  Linear Heat Pipe : Subsystem  AncestorBlock=PlantUtilityBlockset_lib/Hydraulic/Linear Heat Pipe
      mask Display:
      | plot([-1:0.2:1], [1 .8 .6 .5 .5 .5 .5 .5 .6 .8 1])
      | plot([-1:0.2:1], -[1 .8 .6 .5 .5 .5 .5 .5 .6 .8 1])
  Linear Heat Pipe1 : Subsystem  AncestorBlock=PlantUtilityBlockset_lib/Hydraulic/Linear Heat Pipe
      mask Display:
      | plot([-1:0.2:1], [1 .8 .6 .5 .5 .5 .5 .5 .6 .8 1])
      | plot([-1:0.2:1], -[1 .8 .6 .5 .5 .5 .5 .5 .6 .8 1])
  out1 : Outport
  out2 : Outport  Port=2
  wires:
  in1/1 -> Bus Selector/1
  in2/1 -> Linear Heat Pipe1/1(pT_in)
  Linear Heat Pipe1/1(pT_out) -> Bus Creator/1  "p"
  Linear Heat Pipe/1(pT_out) -> Bus Creator1/1  "p"
  Bus Selector/1 -> Linear Heat Pipe/1(pT_in)  "<p>"
  Bus Selector/2 -> Bus Creator/2, Bus Creator1/2  "<T>"
  Bus Creator/1 -> out2/1
  Bus Creator1/1 -> out1/1

== system Simple_lib/Hydraulic/Accumulator ==
  1/I : Gain  Gain=1/2
  Discrete-Time Integrator1 : DiscreteIntegrator  gainval=1  SampleTime=Ts  ICPrevOutput=DiscIntNeverNeededParam  ICPrevScaledInput=DiscIntNeverNeededParam
  Duplex : Subsystem  Tag=Driveline  AncestorBlock=PlantUtilityBlockset_lib/Utility/Duplex  InitFcn=initDuplex
      mask Display:
      | color('white')
      | plot([0 3], [2 2])
      | plot([0 3], [-2 -2])
      | color('black')
      | 
      | plot([0 1 1], [0 0 0.4])
      | plot([1 1 3], [0.6 1 1])
      | plot([1 3 2 1 0 2], [0.6 0.6 0.4 0.6 0.4 0.4])
      | patch([0 2 1],[0.4 0.4 0.6],[0,0,0])
      | plot([3 2 2], [1 1 0.6])
      | plot([2 2 3], [0.4 -1 -1])
  Out1 : Outport
  wires:
  Discrete-Time Integrator1/1 -> Duplex/1(InPot)
  1/I/1 -> Discrete-Time Integrator1/1
  Duplex/1(OutPot) -> Out1/1
  Duplex/2(OutFlow) -> 1/I/1

== system Simple_lib/Hydraulic/Atmosphere ==
  Ambient Pressure : Constant  Value=1e5
  Duplex : PlantUtilityBlockset_lib/Utility/Pull  Tag=Electrical  SystemSampleTime=-1
  Terminator : Terminator
  Out1 : Outport
  wires:
  Duplex/1 -> Out1/1
  Ambient Pressure/1 -> Duplex/1
  Duplex/2 -> Terminator/1

== system Simple_lib/Hydraulic/Heat Sink ==
  pT_in : Inport
  T_in : Inport  Port=2
  Linear Heat Pipe1 : Subsystem
      mask Display:
      | plot([-1:0.2:1], [1 .8 .6 .5 .5 .5 .5 .5 .6 .8 1])
      | plot([-1:0.2:1], -[1 .8 .6 .5 .5 .5 .5 .5 .6 .8 1])
  Linear Heat Pipe2 : Subsystem
      mask Display:
      | plot([-1:0.2:1], [1 .8 .6 .5 .5 .5 .5 .5 .6 .8 1])
      | plot([-1:0.2:1], -[1 .8 .6 .5 .5 .5 .5 .5 .6 .8 1])
  Linear Heat Pipe3 : Subsystem
      mask Display:
      | plot([-1:0.2:1], [1 .8 .6 .5 .5 .5 .5 .5 .6 .8 1])
      | plot([-1:0.2:1], -[1 .8 .6 .5 .5 .5 .5 .5 .6 .8 1])
  R1 : Subsystem  AncestorBlock=PlantUtilityBlockset_lib/Thermal/R17  mask{R=10}
      mask prompts: R "Resistance"
      mask Display:
      | color('white')
      | plot([-1 1 1 -1 -1], [-1 -1 1 1 -1])
      | color('red')
      | patch( [ -1 1 1 -1 -1],[-.51 -.51  -.49 -.49 -.51],[0.85 0 0])
      | patch( [ -1 1 1 -1 -1],[ .51  .51   .49  .49  .51],[0.85 0 0])
      | plot( [ .6 1],[-.5 .2])
      | plot( [ .3 .8],[-.5 .5])
      | plot( [ .0 .5],[-.5 .5])
      | plot( [-.3 .2],[-.5 .5])
      | plot( [-.6 -.1],[-.5 .5])
      | plot( [-.9 -.4],[-.5 .5])
      | plot( [-1 -.7],[-.1 .5])
      | %plot( [ -1 0 1 0 -1 0 1 0 -1 0 1 0 -1],[-6:6]/12)
  R2 : PlantUtilityBlockset_lib/Hydraulic/Heat Sink/R1  R=10
  R3 : PlantUtilityBlockset_lib/Hydraulic/Heat Sink/R1  R=10
  pT_out : Outport
  wires:
  pT_in/1 -> Linear Heat Pipe1/1(pT_in)
  Linear Heat Pipe1/1(pT_out) -> Linear Heat Pipe2/1(pT_in)
  Linear Heat Pipe2/1(pT_out) -> Linear Heat Pipe3/1(pT_in)
  Linear Heat Pipe3/1(pT_out) -> pT_out/1
  T_in/1 -> R3/1, R2/1, R1/1(In1)
  Linear Heat Pipe1/2(T_out) -> R1/2(In2)
  Linear Heat Pipe2/2(T_out) -> R2/2
  Linear Heat Pipe3/2(T_out) -> R3/2

== system Simple_lib/Hydraulic/Isothermal Accumulator ==
  1/I : Gain  Gain=1/2
  Discrete-Time Integrator1 : DiscreteIntegrator  gainval=1  SampleTime=Ts  ICPrevOutput=DiscIntNeverNeededParam  ICPrevScaledInput=DiscIntNeverNeededParam
  Duplex : Subsystem  Tag=Driveline  AncestorBlock=PlantUtilityBlockset_lib/Utility/Duplex  InitFcn=initDuplex
      mask Display:
      | color('white')
      | plot([0 3], [2 2])
      | plot([0 3], [-2 -2])
      | color('black')
      | 
      | plot([0 1 1], [0 0 0.4])
      | plot([1 1 3], [0.6 1 1])
      | plot([1 3 2 1 0 2], [0.6 0.6 0.4 0.6 0.4 0.4])
      | patch([0 2 1],[0.4 0.4 0.6],[0,0,0])
      | plot([3 2 2], [1 1 0.6])
      | plot([2 2 3], [0.4 -1 -1])
  Out1 : Outport
  wires:
  Discrete-Time Integrator1/1 -> Duplex/1(InPot)
  1/I/1 -> Discrete-Time Integrator1/1
  Duplex/1(OutPot) -> Out1/1
  Duplex/2(OutFlow) -> 1/I/1

== system Simple_lib/Hydraulic/Isothermal Pump ==
  P : Inport
  w : Inport  Port=2
  T : Inport  Port=3
  Area : Gain
  Area1 : Gain  Gain=-1
  Area3 : Gain  Gain=-1
  PushBack : Subsystem  AncestorBlock=PlantUtilityBlockset_lib/Utility/Push  InitFcn=initSimplex
      mask Display:
      | color('white')
      | plot([0 3], [2 2])
      | plot([0 3], [-2 -2])
      | color('black')
      | 
      | plot([0 2 2 3], [1 1 0 0])
      | plot([1 3 2 1 0 2], [0.6 0.6 0.4 0.6 0.4 0.4])
      | patch([1 3 2],[0.6 0.6 0.4],[0,0,0])
      | plot([0 1 1], [1 1 0.6])
      | plot([1 1 0], [0.4 -1 -1])
  PushBack1 : Subsystem  AncestorBlock=PlantUtilityBlockset_lib/Utility/Push  InitFcn=initSimplex
      mask Display:
      | color('white')
      | plot([0 3], [2 2])
      | plot([0 3], [-2 -2])
      | color('black')
      | 
      | plot([0 2 2 3], [1 1 0 0])
      | plot([1 3 2 1 0 2], [0.6 0.6 0.4 0.6 0.4 0.4])
      | patch([1 3 2],[0.6 0.6 0.4],[0,0,0])
      | plot([0 1 1], [1 1 0.6])
      | plot([1 1 0], [0.4 -1 -1])
  PushBack2 : Subsystem  AncestorBlock=PlantUtilityBlockset_lib/Utility/Push  InitFcn=initSimplex
      mask Display:
      | color('white')
      | plot([0 3], [2 2])
      | plot([0 3], [-2 -2])
      | color('black')
      | 
      | plot([0 2 2 3], [1 1 0 0])
      | plot([1 3 2 1 0 2], [0.6 0.6 0.4 0.6 0.4 0.4])
      | patch([1 3 2],[0.6 0.6 0.4],[0,0,0])
      | plot([0 1 1], [1 1 0.6])
      | plot([1 1 0], [0.4 -1 -1])
  Sum : Sum  Inputs=+|+
  VolPerRad : Gain
  wires:
  VolPerRad/1 -> Area3/1, PushBack1/2(InFlow)
  Area3/1 -> PushBack/2(InFlow)
  PushBack2/1(OutPot) -> VolPerRad/1
  Area1/1 -> Sum/2
  Area/1 -> PushBack2/2(InFlow)
  Sum/1 -> Area/1
  PushBack1/1(OutPot) -> Area1/1
  PushBack/1(OutPot) -> Sum/1
  T/1 -> PushBack1/1(InPot)
  P/1 -> PushBack/1(InPot)
  w/1 -> PushBack2/1(InPot)

== system Simple_lib/Hydraulic/Isothermal Tank ==
  Ambient Pressure : Constant  Value=1e5
  Duplex : PlantUtilityBlockset_lib/Utility/Pull  Tag=Electrical  SystemSampleTime=-1
  Terminator : Terminator
  Out1 : Outport
  wires:
  Duplex/1 -> Out1/1
  Ambient Pressure/1 -> Duplex/1
  Duplex/2 -> Terminator/1

== system Simple_lib/Hydraulic/Linear Heat Pipe ==
  note: \Delta T = Q / (qc\rho))
  note: \Delta p = - k q
  pT_in : Inport
  Bus Creator1 : BusCreator  Inputs=2
  Bus Selector : BusSelector  OutputSignals=T,p
  Gain : Gain  Gain=-1
  Gain1 : Gain  Gain=1e3
  Product : Product  Inputs=*///
  Pull : Subsystem  Tag=Electrical  AncestorBlock=PlantUtilityBlockset_lib/Utility/Pull  InitFcn=initDuplex
      mask Display:
      | color('white')
      | plot([0 3], [2 2])
      | plot([0 3], [-2 -2])
      | color('black')
      | 
      | plot([0 1 1], [0 0 0.4])
      | plot([1 1 3], [0.6 1 1])
      | plot([1 3 2 1 0 2], [0.6 0.6 0.4 0.6 0.4 0.4])
      | patch([0 2 1],[0.4 0.4 0.6],[0,0,0])
      | plot([3 2 2], [1 1 0.6])
      | plot([2 2 3], [0.4 -1 -1])
  Pull1 : PlantUtilityBlockset_lib/Hydraulic/Linear Heat Pipe/Pull  Tag=Electrical  SystemSampleTime=-1
  Push : Subsystem  AncestorBlock=PlantUtilityBlockset_lib/Utility/Push  InitFcn=initSimplex
      mask Display:
      | color('white')
      | plot([0 3], [2 2])
      | plot([0 3], [-2 -2])
      | color('black')
      | 
      | plot([0 2 2 3], [1 1 0 0])
      | plot([1 3 2 1 0 2], [0.6 0.6 0.4 0.6 0.4 0.4])
      | patch([1 3 2],[0.6 0.6 0.4],[0,0,0])
      | plot([0 1 1], [1 1 0.6])
      | plot([1 1 0], [0.4 -1 -1])
  Sum : Sum  Inputs=|++
  Sum1 : Sum  Inputs=++|
  c : Constant  Value=4200
  rho : Constant  Value=1000
  pT_out : Outport
  T_out : Outport  Port=2
  wires:
  Push/1(OutPot) -> Bus Selector/1
  Sum/1 -> Bus Creator1/2  "p"
  Gain/1 -> Sum/2
  Pull/2(OutFlow) -> Push/2(InFlow), Gain1/1, Product/2  "q"
  Gain1/1 -> Gain/1
  Pull/1(OutPot) -> pT_out/1
  pT_in/1 -> Push/1(InPot)
  Bus Selector/2 -> Sum/1  "<p>"
  Bus Creator1/1 -> Pull/1(InPot)
  Pull1/1 -> T_out/1  "T"
  Bus Selector/1 -> Sum1/2, Pull1/1  "<T>"
  Sum1/1 -> Bus Creator1/1  "T"
  Product/1 -> Sum1/1
  Pull1/2 -> Product/1
  c/1 -> Product/3
  rho/1 -> Product/4

== system Simple_lib/Hydraulic/Linear Pipe ==
  pT_in : Inport
  Gain : Gain  Gain=-1
  Gain1 : Gain  Gain=1e3
  Pull : Subsystem  Tag=Electrical  AncestorBlock=PlantUtilityBlockset_lib/Utility/Pull  InitFcn=initDuplex
      mask Display:
      | color('white')
      | plot([0 3], [2 2])
      | plot([0 3], [-2 -2])
      | color('black')
      | 
      | plot([0 1 1], [0 0 0.4])
      | plot([1 1 3], [0.6 1 1])
      | plot([1 3 2 1 0 2], [0.6 0.6 0.4 0.6 0.4 0.4])
      | patch([0 2 1],[0.4 0.4 0.6],[0,0,0])
      | plot([3 2 2], [1 1 0.6])
      | plot([2 2 3], [0.4 -1 -1])
  Push : Subsystem  AncestorBlock=PlantUtilityBlockset_lib/Utility/Push  InitFcn=initSimplex
      mask Display:
      | color('white')
      | plot([0 3], [2 2])
      | plot([0 3], [-2 -2])
      | color('black')
      | 
      | plot([0 2 2 3], [1 1 0 0])
      | plot([1 3 2 1 0 2], [0.6 0.6 0.4 0.6 0.4 0.4])
      | patch([1 3 2],[0.6 0.6 0.4],[0,0,0])
      | plot([0 1 1], [1 1 0.6])
      | plot([1 1 0], [0.4 -1 -1])
  Sum : Sum  Inputs=|++
  pT_out : Outport
  wires:
  Push/1(OutPot) -> Sum/1
  Sum/1 -> Pull/1(InPot)
  Gain/1 -> Sum/2
  Pull/2(OutFlow) -> Push/2(InFlow), Gain1/1
  Gain1/1 -> Gain/1
  Pull/1(OutPot) -> pT_out/1
  pT_in/1 -> Push/1(InPot)

== system Simple_lib/Hydraulic/Motor ==
  ctrl : Inport
  Characterisation : Lookup_n-D  BreakpointsForDimension1=[1:3]  BreakpointsForDimension2=[1:3]  RndMeth=Simplest  InputSameDT=on
  Inertia : Subsystem  AncestorBlock=PlantUtilityBlockset_lib/Driveline/InertialState
      mask Display:
      | color('white');
      | plot([-1 4],[1 1]);
      | plot([-1 4],[-1 -1]);
      | color('black')
      | plot([1 4],[0 0]);
      | plot([-1 -.9 -.5 0 .5 .9 1  .9  .5  0 -.5 -.9 -1],      [ 0  .5 .9 1 .9 .5 0 -.5 -.9 -1 -.9 -.5  0]);
      | plot([4 4.5 4.5 4],[0 -0.25 0.25 0])
  PushBack : Subsystem  AncestorBlock=PlantUtilityBlockset_lib/Utility/Push  InitFcn=initSimplex
      mask Display:
      | color('white')
      | plot([0 3], [2 2])
      | plot([0 3], [-2 -2])
      | color('black')
      | 
      | plot([0 2 2 3], [1 1 0 0])
      | plot([1 3 2 1 0 2], [0.6 0.6 0.4 0.6 0.4 0.4])
      | patch([1 3 2],[0.6 0.6 0.4],[0,0,0])
      | plot([0 1 1], [1 1 0.6])
      | plot([1 1 0], [0.4 -1 -1])
  w : Outport
  wires:
  Characterisation/1 -> PushBack/2(InFlow)  "torque"
  PushBack/1(OutPot) -> Characterisation/1  "speed"
  ctrl/1 -> Characterisation/2
  Inertia/1(Out1) -> w/1, PushBack/1(InPot)

== system Simple_lib/Hydraulic/Pressure Meter ==
  note: NOTE: Does not necessarily need Pushback
  In : Inport
  Ground : Ground
  PushBack : Subsystem  AncestorBlock=PlantUtilityBlockset_lib/Utility/Push  InitFcn=initSimplex
      mask Display:
      | color('white')
      | plot([0 3], [2 2])
      | plot([0 3], [-2 -2])
      | color('black')
      | 
      | plot([0 2 2 3], [1 1 0 0])
      | plot([1 3 2 1 0 2], [0.6 0.6 0.4 0.6 0.4 0.4])
      | patch([1 3 2],[0.6 0.6 0.4],[0,0,0])
      | plot([0 1 1], [1 1 0.6])
      | plot([1 1 0], [0.4 -1 -1])
  p : Outport
  wires:
  In/1 -> PushBack/1(InPot)
  PushBack/1(OutPot) -> p/1
  Ground/1 -> PushBack/2(InFlow)
